simulink model "circuit_RC"  (R2023b)
settings: Solver=VariableStepAuto  StartTime=0.0  StopTime=10.0  RelTol=1e-3
settings Model: Creator=Mihai  LastModifiedBy=Mihai

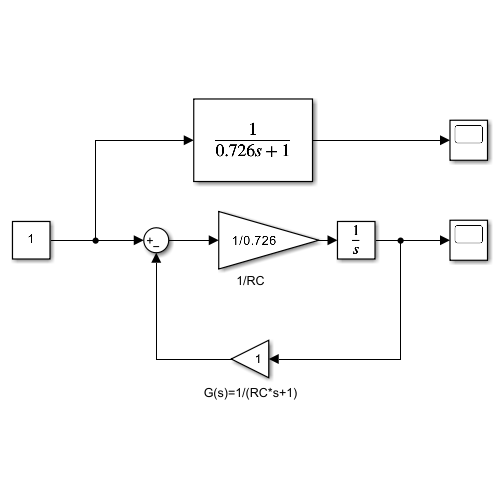
[thumbnail: Simulink's stored preview of the top-level diagram]
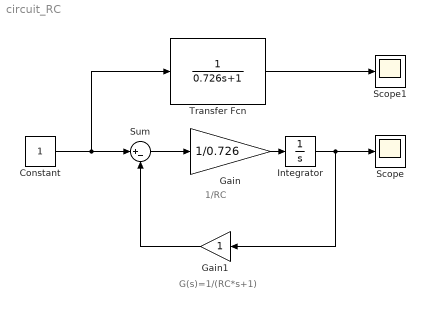
== system circuit_RC ==
  note: 1/RC
  note: G(s)=1/(RC*s+1)
  Constant : Constant
  Gain : Gain  Gain=1/0.726
  Gain1 : Gain
  Integrator : Integrator
  Scope : Scope
  Scope1 : Scope
  Sum : Sum  Inputs=|+-
  Transfer Fcn : TransferFcn  Denominator=[0.726 1]
  wires:
  Gain/1 -> Integrator/1
  Sum/1 -> Gain/1
  Constant/1 -> Transfer Fcn/1, Sum/1
  Gain1/1 -> Sum/2
  Integrator/1 -> Scope/1, Gain1/1
  Transfer Fcn/1 -> Scope1/1
